simulink model "GenOptRockerMomtryDisHndlr"  (R2017b)
settings: configuration reference "JD_ConfigsetAUTOSARMulti10msec" (kept outside this file)
values from neighbouring files (symbols this model uses):
  EolDurnLong = AUTOSAR.Parameter    [GenOptRockerMomtryDisHndlr_DD.m]
  EolDurnRetain = AUTOSAR.Parameter    [GORMDH_DD.m]
  EolDurnSho = AUTOSAR.Parameter    [GenOptRockerMomtryDisHndlr_DD.m]
  RMI_Error = Simulink.Parameter    [GORMDH_DD.m]
  Transition_Add = Simulink.Parameter    [GORMDH_DD.m]
  Transition_Count = Simulink.Parameter    [GORMDH_DD.m]
  Transition_Zero = Simulink.Parameter    [GORMDH_DD.m]
undefined symbols (not defined in the file or in its folder): DiagBool, EnCtrlDisSt, EnCtrlSeln, EnCtrlSts
libraries: simulink x3
settings Model: Creator=KIH3CPW  LastModifiedBy=KIH3CPW
settings ConfigSetRef: SourceLocation=Base Workspace

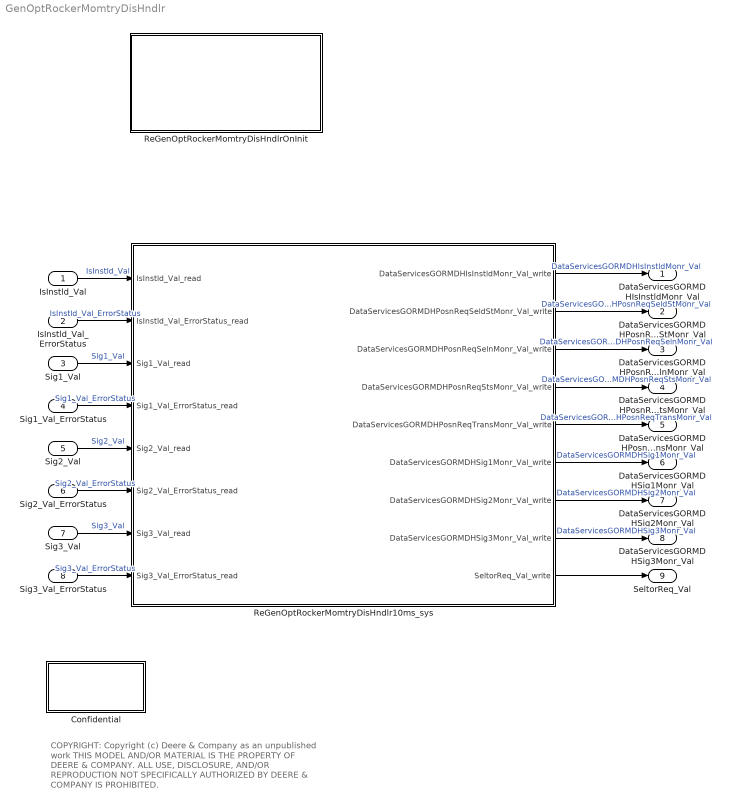
== system GenOptRockerMomtryDisHndlr ==
  note: COPYRIGHT:
      | Copyright (c) Deere & Company as an unpublished work
      | THIS MODEL AND/OR MATERIAL IS THE PROPERTY OF
      | DEERE & COMPANY.  ALL USE, DISCLOSURE, AND/OR
      | REPRODUCTION NOT SPECIFICALLY AUTHORIZED BY
      | DEERE & COMPANY IS PROHIBITED.
  IsInstld_Val : Inport  OutDataTypeStr=Bool  PortDimensions=1
  IsInstld_Val_ErrorStatus : Inport  Port=2  OutDataTypeStr=uint8  PortDimensions=1
  Sig1_Val : Inport  Port=3  OutDataTypeStr=Bool  PortDimensions=1
  Sig1_Val_ErrorStatus : Inport  Port=4  OutDataTypeStr=uint8  PortDimensions=1
  Sig2_Val : Inport  Port=5  OutDataTypeStr=Bool  PortDimensions=1
  Sig2_Val_ErrorStatus : Inport  Port=6  OutDataTypeStr=uint8  PortDimensions=1
  Sig3_Val : Inport  Port=7  OutDataTypeStr=Bool  PortDimensions=1
  Sig3_Val_ErrorStatus : Inport  Port=8  OutDataTypeStr=uint8  PortDimensions=1
  Confidential : Subsystem
      mask Display: image('ConfidentialStamp.jpg')
  ReGenOptRockerMomtryDisHndlr10ms_sys : Subsystem  TreatAsAtomicUnit=on  SystemSampleTime=0.01
  ReGenOptRockerMomtryDisHndlrOnInit : Subsystem
  DataServicesGORMDHIsInstldMonr_Val : Outport  OutDataTypeStr=Enum: DiagBool  PortDimensions=1
  DataServicesGORMDHPosnReqSeldStMonr_Val : Outport  Port=2  OutDataTypeStr=Enum: EnCtrlDisSt  PortDimensions=1
  DataServicesGORMDHPosnReqSelnMonr_Val : Outport  Port=3  OutDataTypeStr=Enum: EnCtrlSeln  PortDimensions=1
  DataServicesGORMDHPosnReqStsMonr_Val : Outport  Port=4  OutDataTypeStr=Enum: EnCtrlSts  PortDimensions=1
  DataServicesGORMDHPosnReqTransMonr_Val : Outport  Port=5  OutDataTypeStr=CntAbsMod  PortDimensions=1
  DataServicesGORMDHSig1Monr_Val : Outport  Port=6  OutDataTypeStr=Enum: DiagBool  PortDimensions=1
  DataServicesGORMDHSig2Monr_Val : Outport  Port=7  OutDataTypeStr=Enum: DiagBool  PortDimensions=1
  DataServicesGORMDHSig3Monr_Val : Outport  Port=8  OutDataTypeStr=Enum: DiagBool  PortDimensions=1
  SeltorReq_Val : Outport  Port=9  OutDataTypeStr=Bus: RecCtrlSelr  PortDimensions=1  BusOutputAsStruct=on
  wires:
  IsInstld_Val/1 -> ReGenOptRockerMomtryDisHndlr10ms_sys/1(IsInstld_Val_read)  "IsInstld_Val"
  IsInstld_Val_ErrorStatus/1 -> ReGenOptRockerMomtryDisHndlr10ms_sys/2(IsInstld_Val_ErrorStatus_read)  "IsInstld_Val_ErrorStatus"
  Sig1_Val/1 -> ReGenOptRockerMomtryDisHndlr10ms_sys/3(Sig1_Val_read)  "Sig1_Val"
  Sig1_Val_ErrorStatus/1 -> ReGenOptRockerMomtryDisHndlr10ms_sys/4(Sig1_Val_ErrorStatus_read)  "Sig1_Val_ErrorStatus"
  Sig2_Val/1 -> ReGenOptRockerMomtryDisHndlr10ms_sys/5(Sig2_Val_read)  "Sig2_Val"
  Sig2_Val_ErrorStatus/1 -> ReGenOptRockerMomtryDisHndlr10ms_sys/6(Sig2_Val_ErrorStatus_read)  "Sig2_Val_ErrorStatus"
  Sig3_Val/1 -> ReGenOptRockerMomtryDisHndlr10ms_sys/7(Sig3_Val_read)  "Sig3_Val"
  Sig3_Val_ErrorStatus/1 -> ReGenOptRockerMomtryDisHndlr10ms_sys/8(Sig3_Val_ErrorStatus_read)  "Sig3_Val_ErrorStatus"
  ReGenOptRockerMomtryDisHndlr10ms_sys/1(DataServicesGORMDHIsInstldMonr_Val_write) -> DataServicesGORMDHIsInstldMonr_Val/1  "DataServicesGORMDHIsInstldMonr_Val"
  ReGenOptRockerMomtryDisHndlr10ms_sys/2(DataServicesGORMDHPosnReqSeldStMonr_Val_write) -> DataServicesGORMDHPosnReqSeldStMonr_Val/1  "DataServicesGORMDHPosnReqSeldStMonr_Val"
  ReGenOptRockerMomtryDisHndlr10ms_sys/3(DataServicesGORMDHPosnReqSelnMonr_Val_write) -> DataServicesGORMDHPosnReqSelnMonr_Val/1  "DataServicesGORMDHPosnReqSelnMonr_Val"
  ReGenOptRockerMomtryDisHndlr10ms_sys/4(DataServicesGORMDHPosnReqStsMonr_Val_write) -> DataServicesGORMDHPosnReqStsMonr_Val/1  "DataServicesGORMDHPosnReqStsMonr_Val"
  ReGenOptRockerMomtryDisHndlr10ms_sys/5(DataServicesGORMDHPosnReqTransMonr_Val_write) -> DataServicesGORMDHPosnReqTransMonr_Val/1  "DataServicesGORMDHPosnReqTransMonr_Val"
  ReGenOptRockerMomtryDisHndlr10ms_sys/6(DataServicesGORMDHSig1Monr_Val_write) -> DataServicesGORMDHSig1Monr_Val/1  "DataServicesGORMDHSig1Monr_Val"
  ReGenOptRockerMomtryDisHndlr10ms_sys/7(DataServicesGORMDHSig2Monr_Val_write) -> DataServicesGORMDHSig2Monr_Val/1  "DataServicesGORMDHSig2Monr_Val"
  ReGenOptRockerMomtryDisHndlr10ms_sys/8(DataServicesGORMDHSig3Monr_Val_write) -> DataServicesGORMDHSig3Monr_Val/1  "DataServicesGORMDHSig3Monr_Val"
  ReGenOptRockerMomtryDisHndlr10ms_sys/9(SeltorReq_Val_write) -> SeltorReq_Val/1

== system GenOptRockerMomtryDisHndlr/Confidential ==

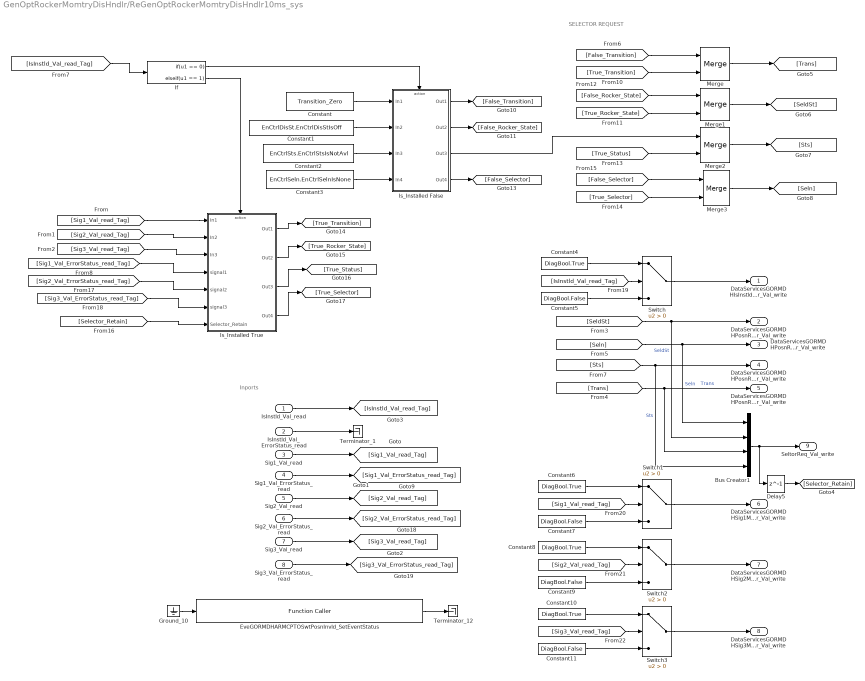
== system GenOptRockerMomtryDisHndlr/ReGenOptRockerMomtryDisHndlr10ms_sys ==
  note: SELECTOR REQUEST
  note: Inports
  IsInstld_Val_read : Inport
  IsInstld_Val_ErrorStatus_read : Inport  Port=2
  Sig1_Val_read : Inport  Port=3
  Sig1_Val_ErrorStatus_read : Inport  Port=4
  Sig2_Val_read : Inport  Port=5
  Sig2_Val_ErrorStatus_read : Inport  Port=6
  Sig3_Val_read : Inport  Port=7
  Sig3_Val_ErrorStatus_read : Inport  Port=8
  Bus Creator1 : BusCreator  Inputs=4  OutDataTypeStr=Bus: RecCtrlSelr
  Constant : Constant  Value=Transition_Zero  OutDataTypeStr=CntAbsMod
  Constant1 : Constant  Value=EnCtrlDisSt.EnCtrlDisStIsOff
  Constant{4,6,8,10} (4 alike) : Constant  Value=DiagBool.True
  Constant{5,7,9,11} (4 alike) : Constant  Value=DiagBool.False
  Constant2 : Constant  Value=EnCtrlSts.EnCtrlStsIsNotAvl
  Constant3 : Constant  Value=EnCtrlSeln.EnCtrlSelnIsNone
  Delay5 : Delay  DelayLength=1  InitialCondition=0
  EveGORMDHARMCPTOSwtPosnInvld_SetEventStatus : FunctionCaller  Description=API for SWCs to report a monitor result to the Dem.This function is reentrant (for different EventId).This function is not reentrant with the other operations defined in DiagnosticMonitor (for the same EventId)This function is synchronous.  FunctionPrototype=ERR = EveGORMDHARMCPTOSwtPosnInvld_SetEventStatus(EventStatus)  InputArgumentSpecifications=Dem_EventStatusType.DEM_EVENT_STATUS_PASSED  OutputArgumentSpecifications=P_Std_ReturnType
  Ground_10 : Ground
  If : If  IfExpression=u1 == 0  ElseIfExpressions=u1 == 1  ShowElse=off
  Is_Installed False : Subsystem  TreatAsAtomicUnit=on
  Is_Installed True : Subsystem  TreatAsAtomicUnit=on
  Merge{,1..3} (4 alike) : Merge
  Switch{,1..3} (4 alike) : Switch  Criteria=u2 > Threshold
  Terminator_1 : Terminator
  Terminator_12 : Terminator
  DataServicesGORMDHIsInstldMonr_Val_write : Outport
  DataServicesGORMDHPosnReqSeldStMonr_Val_write : Outport  Port=2
  DataServicesGORMDHPosnReqSelnMonr_Val_write : Outport  Port=3
  DataServicesGORMDHPosnReqStsMonr_Val_write : Outport  Port=4
  DataServicesGORMDHPosnReqTransMonr_Val_write : Outport  Port=5
  DataServicesGORMDHSig1Monr_Val_write : Outport  Port=6
  DataServicesGORMDHSig2Monr_Val_write : Outport  Port=7
  DataServicesGORMDHSig3Monr_Val_write : Outport  Port=8
  SeltorReq_Val_write : Outport  Port=9  OutDataTypeStr=Bus: RecCtrlSelr
  wires:
  Switch/1 -> DataServicesGORMDHIsInstldMonr_Val_write/1
  Switch1/1 -> DataServicesGORMDHSig1Monr_Val_write/1
  Switch2/1 -> DataServicesGORMDHSig2Monr_Val_write/1
  Switch3/1 -> DataServicesGORMDHSig3Monr_Val_write/1
  IsInstld_Val_ErrorStatus_read/1 -> Terminator_1/1
  Sig1_Val_read/1 -> [Sig1_Val_read_Tag]
  Sig1_Val_ErrorStatus_read/1 -> [Sig1_Val_ErrorStatus_read_Tag]
  Sig2_Val_read/1 -> [Sig2_Val_read_Tag]
  Sig2_Val_ErrorStatus_read/1 -> [Sig2_Val_ErrorStatus_read_Tag]
  Sig3_Val_read/1 -> [Sig3_Val_read_Tag]
  Sig3_Val_ErrorStatus_read/1 -> [Sig3_Val_ErrorStatus_read_Tag]
  Ground_10/1 -> EveGORMDHARMCPTOSwtPosnInvld_SetEventStatus/1
  EveGORMDHARMCPTOSwtPosnInvld_SetEventStatus/1 -> Terminator_12/1
  [Sig1_Val_read_Tag] -> Is_Installed True/1(In1)
  [Sig2_Val_read_Tag] -> Is_Installed True/2(In2)
  [Sig3_Val_read_Tag] -> Is_Installed True/3(In3)
  IsInstld_Val_read/1 -> [IsInstld_Val_read_Tag]
  Merge/1 -> [Trans]
  Merge1/1 -> [SeldSt]
  Merge2/1 -> [Sts]
  Is_Installed True/1(Out1) -> [True_Transition]
  Is_Installed True/2(Out2) -> [True_Rocker_State]
  Is_Installed True/4(Out4) -> [True_Selector]
  [False_Transition] -> Merge/1
  [False_Rocker_State] -> Merge1/1
  [True_Rocker_State] -> Merge1/2
  Is_Installed False/3(Out3) -> Merge2/1
  [False_Selector] -> Merge3/1
  [True_Selector] -> Merge3/2
  [IsInstld_Val_read_Tag] -> If/1
  If/1 -> Is_Installed False/Action
  Constant/1 -> Is_Installed False/1(In1)
  Constant1/1 -> Is_Installed False/2(In2)
  Constant2/1 -> Is_Installed False/3(In3)
  Constant3/1 -> Is_Installed False/4(In4)
  Is_Installed False/1(Out1) -> [False_Transition]
  Is_Installed False/2(Out2) -> [False_Rocker_State]
  Is_Installed False/4(Out4) -> [False_Selector]
  If/2 -> Is_Installed True/Action
  Constant4/1 -> Switch/1
  Constant5/1 -> Switch/3
  [IsInstld_Val_read_Tag] -> Switch/2
  [Sig1_Val_read_Tag] -> Switch1/2
  Constant7/1 -> Switch1/3
  Constant6/1 -> Switch1/1
  [Sig2_Val_read_Tag] -> Switch2/2
  Constant8/1 -> Switch2/1
  Constant9/1 -> Switch2/3
  [Sig3_Val_read_Tag] -> Switch3/2
  Constant10/1 -> Switch3/1
  Constant11/1 -> Switch3/3
  Merge3/1 -> [Seln]
  Delay5/1 -> [Selector_Retain]
  Bus Creator1/1 -> SeltorReq_Val_write/1, Delay5/1
  [Sts] -> Bus Creator1/4, DataServicesGORMDHPosnReqStsMonr_Val_write/1  "Sts"
  [Trans] -> Bus Creator1/3, DataServicesGORMDHPosnReqTransMonr_Val_write/1  "Trans"
  [Seln] -> Bus Creator1/1, DataServicesGORMDHPosnReqSelnMonr_Val_write/1  "Seln"
  [SeldSt] -> Bus Creator1/2, DataServicesGORMDHPosnReqSeldStMonr_Val_write/1  "SeldSt"
  [Sig1_Val_ErrorStatus_read_Tag] -> Is_Installed True/4(signal1)
  [Sig3_Val_ErrorStatus_read_Tag] -> Is_Installed True/6("signal3 ")
  Is_Installed True/3(Out3) -> [True_Status]
  [True_Status] -> Merge2/2
  [Selector_Retain] -> Is_Installed True/7(Selector_Retain)
  [Sig2_Val_ErrorStatus_read_Tag] -> Is_Installed True/5(signal2)
  [True_Transition] -> Merge/2

== system GenOptRockerMomtryDisHndlr/ReGenOptRockerMomtryDisHndlrOnInit ==
  Event Listener : EventListener  EventType=Initialize  EventName=reset  VariantControl=Variant

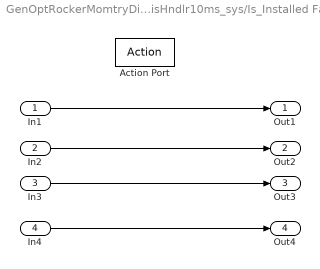
== system GenOptRockerMomtryDisHndlr/ReGenOptRockerMomtryDisHndlr10ms_sys/Is_Installed False ==
  In1 : Inport
  In2 : Inport  Port=2
  In3 : Inport  Port=3
  In4 : Inport  Port=4
  Action Port : ActionPort  ActionType=then
  Out1 : Outport
  Out2 : Outport  Port=2
  Out3 : Outport  Port=3
  Out4 : Outport  Port=4
  wires:
  In1/1 -> Out1/1
  In4/1 -> Out4/1
  In3/1 -> Out3/1
  In2/1 -> Out2/1

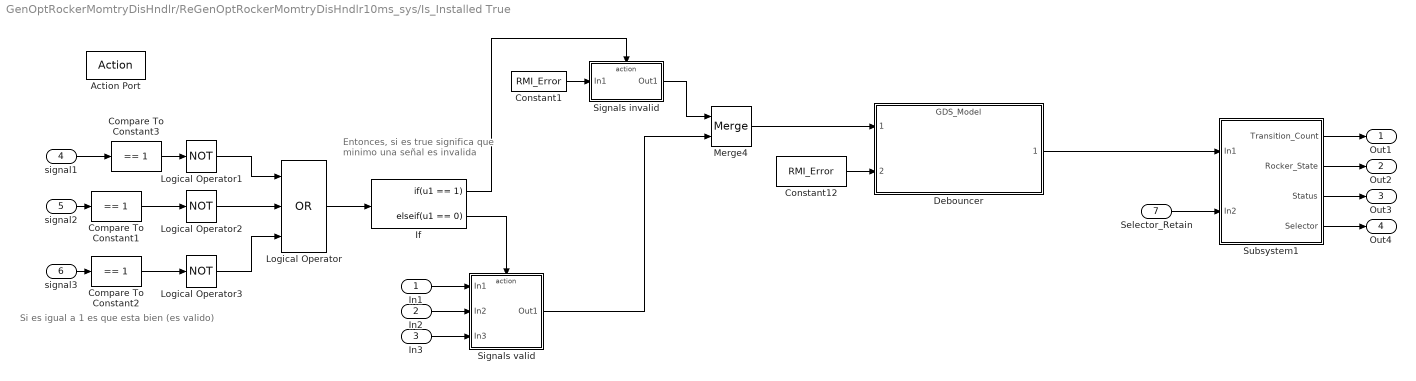
== system GenOptRockerMomtryDisHndlr/ReGenOptRockerMomtryDisHndlr10ms_sys/Is_Installed True ==
  note: Si es igual a 1 es que esta bien (es valido)
  note: Entonces, si es true significa que minimo una señal es invalida
  In1 : Inport
  In2 : Inport  Port=2
  In3 : Inport  Port=3
  signal1 : Inport  Port=4
  signal2 : Inport  Port=5
  "signal3 " : Inport  Port=6
  Selector_Retain : Inport  Port=7
  Action Port : ActionPort  ActionType=elseif
  Compare To Constant1 : simulink/Logic and Bit Operations/Compare To Constant  relop===  const=1  OutDataTypeStr=boolean
  Compare To Constant2 : simulink/Logic and Bit Operations/Compare To Constant  relop===  const=1  OutDataTypeStr=boolean
  Compare To Constant3 : simulink/Logic and Bit Operations/Compare To Constant  relop===  const=1  OutDataTypeStr=boolean
  Constant1 : Constant  Value=RMI_Error
  Constant12 : Constant  Value=RMI_Error
  "Debouncer " : ModelReference  ModelNameDialog=GDS_Model.slx  SimulationMode=Normal  ModelReferenceVersion=1.8
  If : If  IfExpression=u1 == 1  ElseIfExpressions=u1 == 0  ShowElse=off
  Logical Operator : Logic  Operator=OR  Inputs=3  AllPortsSameDT=off  OutDataTypeStr=boolean
  Logical Operator1 : Logic  Operator=NOT  AllPortsSameDT=off  OutDataTypeStr=boolean
  Logical Operator2 : Logic  Operator=NOT  AllPortsSameDT=off  OutDataTypeStr=boolean
  Logical Operator3 : Logic  Operator=NOT  AllPortsSameDT=off  OutDataTypeStr=boolean
  Merge4 : Merge
  Signals invalid : Subsystem  TreatAsAtomicUnit=on
  Signals valid : Subsystem  TreatAsAtomicUnit=on
  Subsystem1 : Subsystem
  Out1 : Outport
  Out2 : Outport  Port=2
  Out3 : Outport  Port=3
  Out4 : Outport  Port=4
  wires:
  In3/1 -> Signals valid/3(In3)
  In2/1 -> Signals valid/2(In2)
  In1/1 -> Signals valid/1(In1)
  Compare To Constant2/1 -> Logical Operator3/1
  Logical Operator2/1 -> Logical Operator/2
  Logical Operator/1 -> If/1
  Logical Operator3/1 -> Logical Operator/3
  Compare To Constant3/1 -> Logical Operator1/1
  signal2/1 -> Compare To Constant1/1
  "signal3 "/1 -> Compare To Constant2/1
  Logical Operator1/1 -> Logical Operator/1
  Compare To Constant1/1 -> Logical Operator2/1
  signal1/1 -> Compare To Constant3/1
  Merge4/1 -> "Debouncer "/1
  Selector_Retain/1 -> Subsystem1/2(In2)
  Constant12/1 -> "Debouncer "/2
  "Debouncer "/1 -> Subsystem1/1(In1)
  Subsystem1/1(Transition_Count) -> Out1/1
  Subsystem1/2(Rocker_State) -> Out2/1
  Subsystem1/3(Status) -> Out3/1
  Subsystem1/4(Selector) -> Out4/1
  If/2 -> Signals valid/Action
  Signals valid/1(Out1) -> Merge4/2
  If/1 -> Signals invalid/Action
  Constant1/1 -> Signals invalid/1(In1)
  Signals invalid/1(Out1) -> Merge4/1

== system GenOptRockerMomtryDisHndlr/ReGenOptRockerMomtryDisHndlr10ms_sys/Is_Installed True/Signals invalid ==
  In1 : Inport
  Action Port : ActionPort  ActionType=then
  Out1 : Outport
  wires:
  In1/1 -> Out1/1

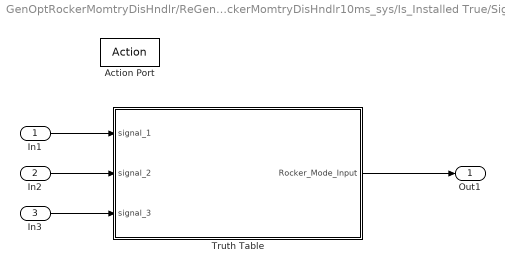
== system GenOptRockerMomtryDisHndlr/ReGenOptRockerMomtryDisHndlr10ms_sys/Is_Installed True/Signals valid ==
  In1 : Inport
  In2 : Inport  Port=2
  In3 : Inport  Port=3
  Action Port : ActionPort  ActionType=elseif
  Truth Table : Truth Table  TreatAsAtomicUnit=on
  Out1 : Outport
  wires:
  In3/1 -> Truth Table/3(signal_3)
  In2/1 -> Truth Table/2(signal_2)
  In1/1 -> Truth Table/1(signal_1)
  Truth Table/1(Rocker_Mode_Input) -> Out1/1

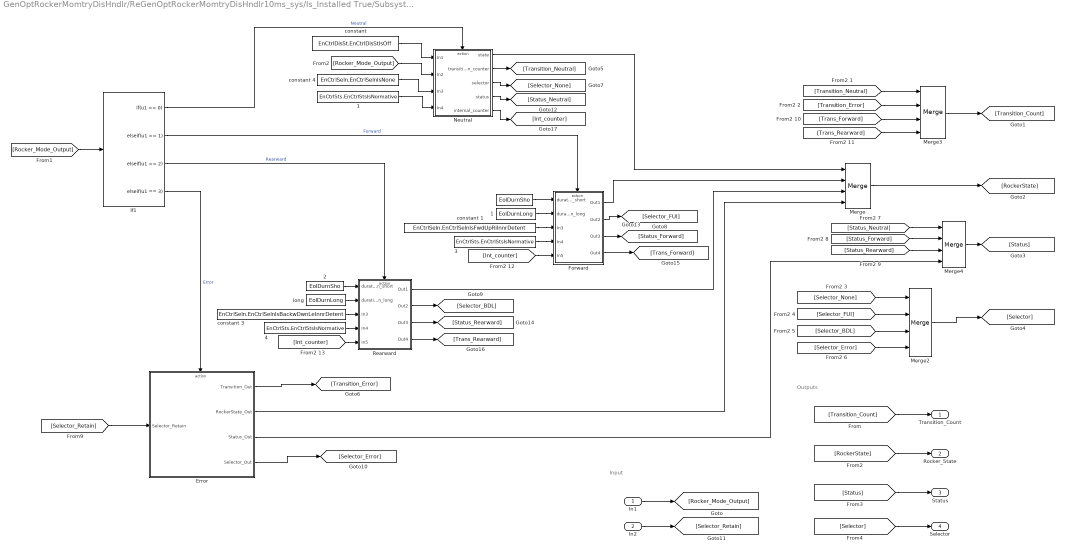
== system GenOptRockerMomtryDisHndlr/ReGenOptRockerMomtryDisHndlr10ms_sys/Is_Installed True/Subsystem1 ==
  note: Outputs
  note: Input
  In1 : Inport
  In2 : Inport  Port=2
  " " : Constant  Value=EolDurnSho
  " 1" : Constant  Value=EolDurnLong
  " 2" : Constant  Value=EolDurnSho
  1 : Constant  Value=EnCtrlSts.EnCtrlStsIsNormative
  3 : Constant  Value=EnCtrlSts.EnCtrlStsIsNormative
  4 : Constant  Value=EnCtrlSts.EnCtrlStsIsNormative
  Error : Subsystem  TreatAsAtomicUnit=on
  Forward : Subsystem  TreatAsAtomicUnit=on
  If1 : If  IfExpression=u1 == 0  ElseIfExpressions=u1 == 1, u1 == 2, u1 == 3  ShowElse=off
  Merge{,2..4} (4 alike) : Merge  Inputs=4
  Neutral : Subsystem  TreatAsAtomicUnit=on
  Rearward : Subsystem  TreatAsAtomicUnit=on
  "constant " : Constant  Value=EnCtrlDisSt.EnCtrlDisStIsOff
  constant 1 : Constant  Value=EnCtrlSeln.EnCtrlSelnIsFwdUpRiInnrDetent
  constant 3 : Constant  Value=EnCtrlSeln.EnCtrlSelnIsBackwDwnLeInnrDetent
  constant 4 : Constant  Value=EnCtrlSeln.EnCtrlSelnIsNone
  long : Constant  Value=EolDurnLong
  Transition_Count : Outport
  Rocker_State : Outport  Port=2
  Status : Outport  Port=3
  Selector : Outport  Port=4
  wires:
  If1/4 -> Error/Action  "Error"
  " "/1 -> Forward/1(duration_short)
  Merge/1 -> [RockerState]
  Neutral/1(state) -> Merge/1
  [Rocker_Mode_Output] -> Neutral/2(In2)
  If1/1 -> Neutral/Action  "Neutral"
  "constant "/1 -> Neutral/1(In1)
  constant 3/1 -> Rearward/3(In3)
  Forward/1(Out1) -> Merge/2
  If1/3 -> Rearward/Action  "Rearward"
  [Rocker_Mode_Output] -> If1/1
  In1/1 -> [Rocker_Mode_Output]
  [Transition_Count] -> Transition_Count/1
  [RockerState] -> Rocker_State/1
  [Status] -> Status/1
  Merge2/1 -> [Selector]
  [Selector] -> Selector/1
  Merge3/1 -> [Transition_Count]
  Merge4/1 -> [Status]
  Error/3(Status_Out) -> Merge4/4
  " 1"/1 -> Forward/2(duration_long)
  constant 4/1 -> Neutral/3(In3)
  constant 1/1 -> Forward/3(In3)
  If1/2 -> Forward/Action  "Forward"
  " 2"/1 -> Rearward/1(duration_short)
  long/1 -> Rearward/2(duration_long)
  Neutral/2(transition_counter) -> [Transition_Neutral]
  Error/1(Transition_Out) -> [Transition_Error]
  [Transition_Error] -> Merge3/2
  [Transition_Neutral] -> Merge3/1
  Neutral/3(selector) -> [Selector_None]
  Forward/2(Out2) -> [Selector_FUI]
  Rearward/2(Out2) -> [Selector_BDL]
  Error/4(Selector_Out) -> [Selector_Error]
  [Selector_None] -> Merge2/1
  [Selector_FUI] -> Merge2/2
  [Selector_BDL] -> Merge2/3
  [Selector_Error] -> Merge2/4
  Rearward/1(Out1) -> Merge/3
  Error/2(RockerState_Out) -> Merge/4
  In2/1 -> [Selector_Retain]
  1/1 -> Neutral/4(In4)
  Neutral/4(status) -> [Status_Neutral]
  3/1 -> Forward/4(In4)
  Forward/3(Out3) -> [Status_Forward]
  4/1 -> Rearward/4(In4)
  Rearward/3(Out3) -> [Status_Rearward]
  [Status_Neutral] -> Merge4/1
  [Status_Forward] -> Merge4/2
  [Status_Rearward] -> Merge4/3
  [Selector_Retain] -> Error/1(Selector_Retain)
  Forward/4(Out4) -> [Trans_Forward]
  [Trans_Forward] -> Merge3/3
  [Trans_Rearward] -> Merge3/4
  [Int_counter] -> Rearward/5(In5)
  Rearward/4(Out4) -> [Trans_Rearward]
  [Int_counter] -> Forward/5(In5)
  Neutral/5(internal_counter) -> [Int_counter]

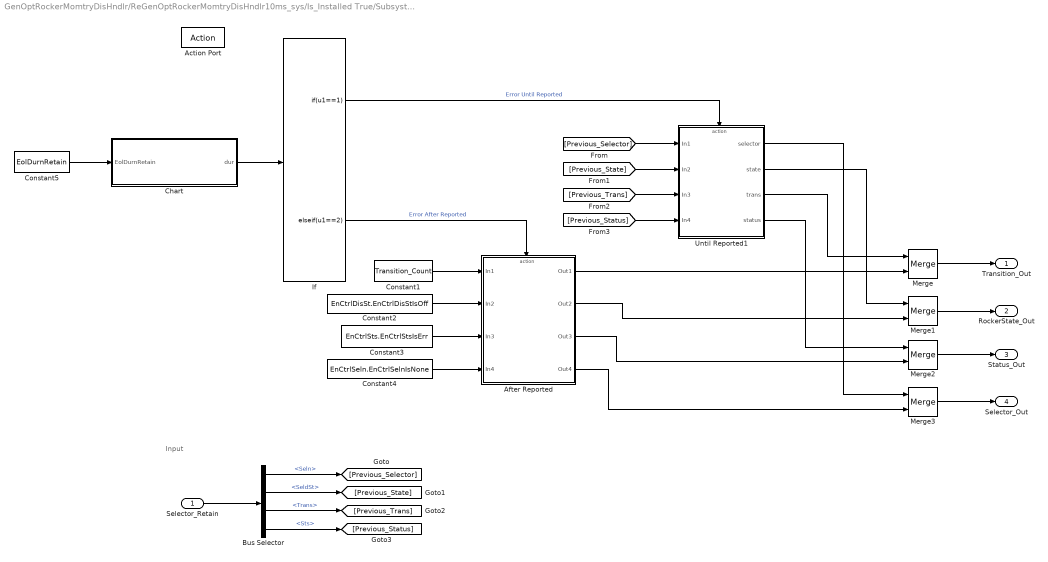
== system GenOptRockerMomtryDisHndlr/ReGenOptRockerMomtryDisHndlr10ms_sys/Is_Installed True/Subsystem1/Error ==
  note: Input
  Selector_Retain : Inport
  Action Port : ActionPort  ActionType=elseif
  After Reported : Subsystem  TreatAsAtomicUnit=on
  Bus Selector : BusSelector  OutputSignals=Seln,SeldSt,Trans,Sts
  Chart : Stateflow chart  TreatAsAtomicUnit=on
  Constant1 : Constant  Value=Transition_Count
  Constant2 : Constant  Value=EnCtrlDisSt.EnCtrlDisStIsOff
  Constant3 : Constant  Value=EnCtrlSts.EnCtrlStsIsErr
  Constant4 : Constant  Value=EnCtrlSeln.EnCtrlSelnIsNone
  Constant5 : Constant  Value=EolDurnRetain
  If : If  IfExpression=u1==1  ElseIfExpressions=u1==2  ShowElse=off
  Merge{,1..3} (4 alike) : Merge
  Until Reported1 : Subsystem  TreatAsAtomicUnit=on
  Transition_Out : Outport
  RockerState_Out : Outport  Port=2
  Status_Out : Outport  Port=3
  Selector_Out : Outport  Port=4
  wires:
  Chart/1(dur) -> If/1
  Constant5/1 -> Chart/1(EolDurnRetain)
  After Reported/3(Out3) -> Merge2/2
  After Reported/2(Out2) -> Merge1/2
  After Reported/4(Out4) -> Merge3/2
  Constant3/1 -> After Reported/3(In3)
  Merge1/1 -> RockerState_Out/1
  After Reported/1(Out1) -> Merge/2
  Constant1/1 -> After Reported/1(In1)
  If/2 -> After Reported/Action  "Error After Reported"
  Merge3/1 -> Selector_Out/1
  Constant4/1 -> After Reported/4(In4)
  If/1 -> Until Reported1/Action  "Error Until Reported"
  Until Reported1/2(state) -> Merge1/1
  Merge/1 -> Transition_Out/1
  Merge2/1 -> Status_Out/1
  Constant2/1 -> After Reported/2(In2)
  Until Reported1/1(selector) -> Merge3/1
  Until Reported1/3(trans) -> Merge/1
  Until Reported1/4(status) -> Merge2/1
  Selector_Retain/1 -> Bus Selector/1
  Bus Selector/1 -> [Previous_Selector]  "<Seln>"
  Bus Selector/2 -> [Previous_State]  "<SeldSt>"
  Bus Selector/3 -> [Previous_Trans]  "<Trans>"
  Bus Selector/4 -> [Previous_Status]  "<Sts>"
  [Previous_Selector] -> Until Reported1/1(In1)
  [Previous_State] -> Until Reported1/2(In2)
  [Previous_Trans] -> Until Reported1/3(In3)
  [Previous_Status] -> Until Reported1/4(In4)

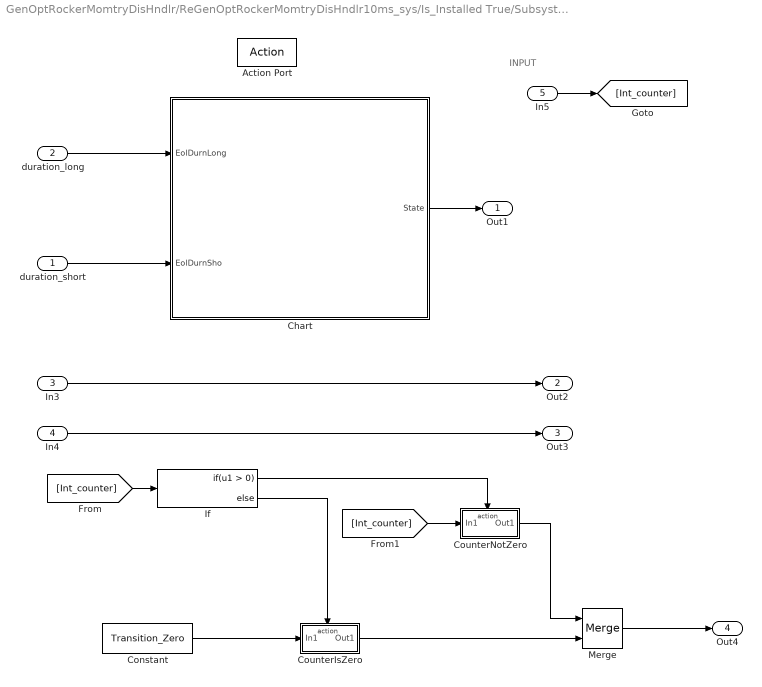
== system GenOptRockerMomtryDisHndlr/ReGenOptRockerMomtryDisHndlr10ms_sys/Is_Installed True/Subsystem1/Forward ==
  note: INPUT
  duration_short : Inport
  duration_long : Inport  Port=2
  In3 : Inport  Port=3
  In4 : Inport  Port=4
  In5 : Inport  Port=5  OutDataTypeStr=CntAbsMod
  Action Port : ActionPort  ActionType=elseif
  Chart : Stateflow chart  TreatAsAtomicUnit=on
  Constant : Constant  Value=Transition_Zero  OutDataTypeStr=CntAbsMod
  CounterIsZero : Subsystem  TreatAsAtomicUnit=on
  CounterNotZero : Subsystem  TreatAsAtomicUnit=on
  If : If
  Merge : Merge
  Out1 : Outport
  Out2 : Outport  Port=2
  Out3 : Outport  Port=3
  Out4 : Outport  Port=4  OutDataTypeStr=CntAbsMod
  wires:
  In3/1 -> Out2/1
  Chart/1(State) -> Out1/1
  In4/1 -> Out3/1
  duration_long/1 -> Chart/1(EolDurnLong)
  duration_short/1 -> Chart/2(EolDurnSho)
  In5/1 -> [Int_counter]
  [Int_counter] -> If/1
  If/1 -> CounterNotZero/Action
  If/2 -> CounterIsZero/Action
  [Int_counter] -> CounterNotZero/1(In1)
  Constant/1 -> CounterIsZero/1(In1)
  CounterIsZero/1(Out1) -> Merge/2
  Merge/1 -> Out4/1
  CounterNotZero/1(Out1) -> Merge/1

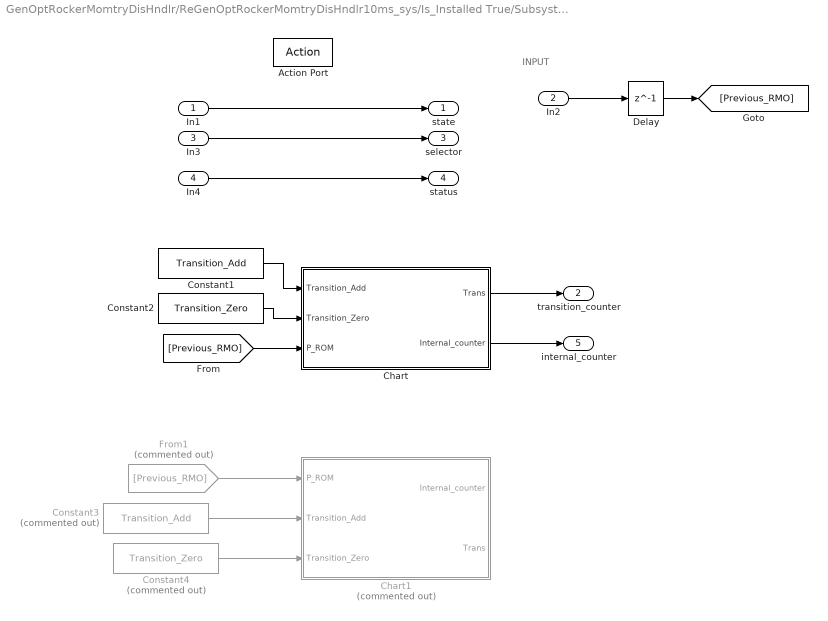
== system GenOptRockerMomtryDisHndlr/ReGenOptRockerMomtryDisHndlr10ms_sys/Is_Installed True/Subsystem1/Neutral ==
  note: INPUT
  In1 : Inport
  In2 : Inport  Port=2
  In3 : Inport  Port=3
  In4 : Inport  Port=4
  Action Port : ActionPort  ActionType=then
  Chart : Stateflow chart  TreatAsAtomicUnit=on
  Chart1 : Stateflow chart  Commented=on  TreatAsAtomicUnit=on
  Constant1 : Constant  Value=Transition_Add
  Constant2 : Constant  Value=Transition_Zero
  Constant3 : Constant  Commented=on  Value=Transition_Add
  Constant4 : Constant  Commented=on  Value=Transition_Zero
  Delay : Delay  DelayLength=1  InitialCondition=0
  From1 : From  Commented=on  GotoTag=Previous_RMO
  state : Outport
  transition_counter : Outport  Port=2  OutDataTypeStr=CntAbsMod
  selector : Outport  Port=3
  status : Outport  Port=4
  internal_counter : Outport  Port=5  OutDataTypeStr=CntAbsMod
  wires:
  In1/1 -> state/1
  Delay/1 -> [Previous_RMO]
  In2/1 -> Delay/1
  In3/1 -> selector/1
  In4/1 -> status/1
  From1/1 -> Chart1/1(P_ROM)
  Constant4/1 -> Chart1/3(Transition_Zero)
  Constant3/1 -> Chart1/2(Transition_Add)
  Constant1/1 -> Chart/1(Transition_Add)
  Constant2/1 -> Chart/2(Transition_Zero)
  [Previous_RMO] -> Chart/3(P_ROM)
  Chart/2(Internal_counter) -> internal_counter/1
  Chart/1(Trans) -> transition_counter/1

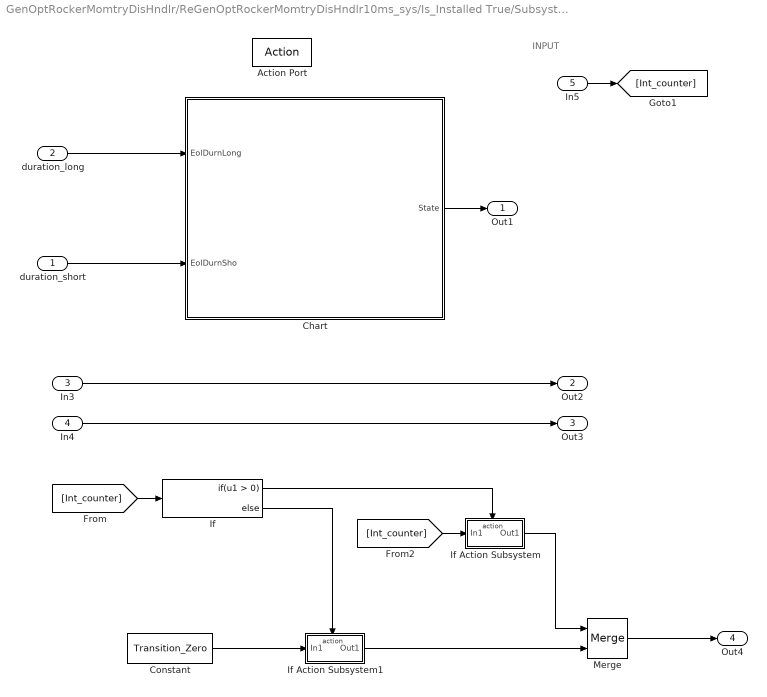
== system GenOptRockerMomtryDisHndlr/ReGenOptRockerMomtryDisHndlr10ms_sys/Is_Installed True/Subsystem1/Rearward ==
  note: INPUT
  duration_short : Inport
  duration_long : Inport  Port=2
  In3 : Inport  Port=3
  In4 : Inport  Port=4
  In5 : Inport  Port=5
  Action Port : ActionPort  ActionType=elseif
  Chart : Stateflow chart  TreatAsAtomicUnit=on
  Constant : Constant  Value=Transition_Zero  OutDataTypeStr=CntAbsMod
  If : If
  If Action Subsystem : Subsystem  TreatAsAtomicUnit=on
  If Action Subsystem1 : Subsystem  TreatAsAtomicUnit=on
  Merge : Merge
  Out1 : Outport
  Out2 : Outport  Port=2
  Out3 : Outport  Port=3
  Out4 : Outport  Port=4  OutDataTypeStr=CntAbsMod
  wires:
  In3/1 -> Out2/1
  Chart/1(State) -> Out1/1
  In4/1 -> Out3/1
  duration_short/1 -> Chart/2(EolDurnSho)
  duration_long/1 -> Chart/1(EolDurnLong)
  If/1 -> If Action Subsystem/Action
  If/2 -> If Action Subsystem1/Action
  Constant/1 -> If Action Subsystem1/1(In1)
  [Int_counter] -> If/1
  [Int_counter] -> If Action Subsystem/1(In1)
  Merge/1 -> Out4/1
  If Action Subsystem/1(Out1) -> Merge/1
  If Action Subsystem1/1(Out1) -> Merge/2
  In5/1 -> [Int_counter]

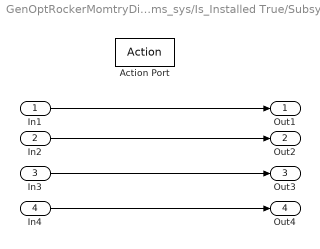
== system GenOptRockerMomtryDisHndlr/ReGenOptRockerMomtryDisHndlr10ms_sys/Is_Installed True/Subsystem1/Error/After Reported ==
  In1 : Inport
  In2 : Inport  Port=2
  In3 : Inport  Port=3
  In4 : Inport  Port=4
  Action Port : ActionPort  ActionType=elseif
  Out1 : Outport
  Out2 : Outport  Port=2
  Out3 : Outport  Port=3
  Out4 : Outport  Port=4
  wires:
  In1/1 -> Out1/1
  In2/1 -> Out2/1
  In3/1 -> Out3/1
  In4/1 -> Out4/1

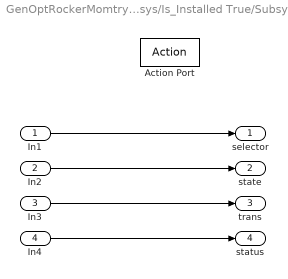
== system GenOptRockerMomtryDisHndlr/ReGenOptRockerMomtryDisHndlr10ms_sys/Is_Installed True/Subsystem1/Error/Until Reported1 ==
  In1 : Inport  OutDataTypeStr=Enum: EnCtrlSeln
  In2 : Inport  Port=2  OutDataTypeStr=Enum: EnCtrlDisSt
  In3 : Inport  Port=3  OutDataTypeStr=CntAbsMod
  In4 : Inport  Port=4  OutDataTypeStr=Enum: EnCtrlSts
  Action Port : ActionPort  ActionType=then
  selector : Outport  OutDataTypeStr=Enum: EnCtrlSeln
  state : Outport  Port=2  OutDataTypeStr=Enum: EnCtrlDisSt
  trans : Outport  Port=3  OutDataTypeStr=CntAbsMod
  status : Outport  Port=4  OutDataTypeStr=Enum: EnCtrlSts
  wires:
  In1/1 -> selector/1
  In2/1 -> state/1
  In3/1 -> trans/1
  In4/1 -> status/1

== system GenOptRockerMomtryDisHndlr/ReGenOptRockerMomtryDisHndlr10ms_sys/Is_Installed True/Subsystem1/Forward/CounterIsZero ==
  In1 : Inport  OutDataTypeStr=CntAbsMod
  Action Port : ActionPort  ActionType=else
  Out1 : Outport  OutDataTypeStr=CntAbsMod
  wires:
  In1/1 -> Out1/1

== system GenOptRockerMomtryDisHndlr/ReGenOptRockerMomtryDisHndlr10ms_sys/Is_Installed True/Subsystem1/Forward/CounterNotZero ==
  In1 : Inport  OutDataTypeStr=CntAbsMod
  Action Port : ActionPort  ActionType=then
  Out1 : Outport  OutDataTypeStr=CntAbsMod
  wires:
  In1/1 -> Out1/1

== system GenOptRockerMomtryDisHndlr/ReGenOptRockerMomtryDisHndlr10ms_sys/Is_Installed True/Subsystem1/Rearward/If Action Subsystem ==
  In1 : Inport
  Action Port : ActionPort  ActionType=then
  Out1 : Outport
  wires:
  In1/1 -> Out1/1

== system GenOptRockerMomtryDisHndlr/ReGenOptRockerMomtryDisHndlr10ms_sys/Is_Installed True/Subsystem1/Rearward/If Action Subsystem1 ==
  In1 : Inport  OutDataTypeStr=CntAbsMod
  Action Port : ActionPort  ActionType=else
  Out1 : Outport  OutDataTypeStr=CntAbsMod
  wires:
  In1/1 -> Out1/1

== matlab function GenOptRockerMomtryDisHndlr/ReGenOptRockerMomtryDisHndlr10ms_sys/Is_Installed True/Signals valid/Truth Table ==
  data: signal_1 input boolean; signal_2 input boolean; Rocker_Mode_Input output double; signal_3 input boolean
function Rocker_Mode_Input = fcn(signal_1, signal_2, signal_3)

aVarTruthTableCondition_1 = false;
aVarTruthTableCondition_2 = false;
aVarTruthTableCondition_3 = false;


% Signal 1

aVarTruthTableCondition_1 = logical(signal_1 == 1);

% Signal 2

aVarTruthTableCondition_2 = logical(signal_2 == 1);

% Signal 3

aVarTruthTableCondition_3 = logical(signal_3 == 1);

if (~aVarTruthTableCondition_1 && ~aVarTruthTableCondition_2 && ~aVarTruthTableCondition_3)
    aFcnTruthTableAction_4();
elseif (~aVarTruthTableCondition_1 && ~aVarTruthTableCondition_2 && aVarTruthTableCondition_3)
    aFcnTruthTableAction_1();
elseif (~aVarTruthTableCondition_1 && aVarTruthTableCondition_2 && ~aVarTruthTableCondition_3)
    aFcnTruthTableAction_4();
elseif (~aVarTruthTableCondition_1 && aVarTruthTableCondition_2 && aVarTruthTableCondition_3)
    aFcnTruthTableAction_4();
elseif (aVarTruthTableCondition_1 && ~aVarTruthTableCondition_2 && ~aVarTruthTableCondition_3)
    aFcnTruthTableAction_3();
elseif (aVarTruthTableCondition_1 && ~aVarTruthTableCondition_2 && aVarTruthTableCondition_3)
    aFcnTruthTableAction_4();
elseif (aVarTruthTableCondition_1 && aVarTruthTableCondition_2 && ~aVarTruthTableCondition_3)
    aFcnTruthTableAction_4();
else % Default
    aFcnTruthTableAction_2();
end

function aFcnTruthTableAction_1()

% Neutral

Rocker_Mode_Input = 0;

function aFcnTruthTableAction_2()

% Forward

Rocker_Mode_Input = 1;

function aFcnTruthTableAction_3()

% Rearward

Rocker_Mode_Input = 2;

function aFcnTruthTableAction_4()

% Error

Rocker_Mode_Input = 3;

== stateflow chart GenOptRockerMomtryDisHndlr/ReGenOptRockerMomtryDisHndlr10ms_sys/Is_Installed True/Subsystem1/Forward/Chart ==
  state On
    during:
    State= EnCtrlDisSt.EnCtrlDisStIsOn;
  state HeldShort
    during:
    State= EnCtrlDisSt.EnCtrlDisStIsHoldSho;
  state HeldLong
    during:
    State= EnCtrlDisSt.EnCtrlDisStIsHoldLong;
  (default) -> On
  On -> HeldShort : [after(EolDurnSho, sec) ]
  HeldShort -> HeldLong : [after(EolDurnLong, sec) ]
  data: State output; EolDurnLong input; EolDurnSho input

== stateflow chart GenOptRockerMomtryDisHndlr/ReGenOptRockerMomtryDisHndlr10ms_sys/Is_Installed True/Subsystem1/Neutral/Chart1 ==
  (default) -> (junction 44) : % trans counter
  (junction 44) -> (junction 45) [order 1] : [P_ROM ==1 || P_ROM==2]
  (junction 44) -> (junction 46) [order 2] : {counter= Transition_Zero + counter; Trans= counter; Internal_counter= counter;}
  (junction 45) -> (junction 47) : {counter= Transition_Zero + counter + Transition_Add; Trans= counter; Internal_counter= counter;}
  (junction 47) -> (junction 46)
  (junction 46) -> (junction 48)
  data: P_ROM input; Transition_Add input; Transition_Zero input; Internal_counter output; Trans output; counter local CntAbsMod [0..255] =Transition_Add

== stateflow chart GenOptRockerMomtryDisHndlr/ReGenOptRockerMomtryDisHndlr10ms_sys/Is_Installed True/Subsystem1/Error/Chart ==
  state Error_Until_Reported
    entry:
    dur=1;
  state Error_After_Reported
    entry:
    dur=2;
  (default) -> Error_Until_Reported
  Error_Until_Reported -> Error_After_Reported : [after(EolDurnRetain,sec) ]
  data: EolDurnRetain input; dur output

== stateflow chart GenOptRockerMomtryDisHndlr/ReGenOptRockerMomtryDisHndlr10ms_sys/Is_Installed True/Subsystem1/Rearward/Chart ==
  state On
    during:
    State= EnCtrlDisSt.EnCtrlDisStIsOn;
  state HeldShort
    during:
    State= EnCtrlDisSt.EnCtrlDisStIsHoldSho;
  state HeldLong
    during:
    State= EnCtrlDisSt.EnCtrlDisStIsHoldLong;
  (default) -> On
  On -> HeldShort : [after(EolDurnSho, sec) ]
  HeldShort -> HeldLong : [after(EolDurnLong, sec) ]
  data: State output; EolDurnLong input; EolDurnSho input

== stateflow chart GenOptRockerMomtryDisHndlr/ReGenOptRockerMomtryDisHndlr10ms_sys/Is_Installed True/Subsystem1/Neutral/Chart ==
  state Transition_Increments
    entry:
    counter= counter + Transition_Add+ Transition_Zero;
    Trans= counter;
    Internal_counter= counter;
  state Transition_Same
    entry:
    counter= Transition_Zero + counter;
    Trans= counter;
    Internal_counter=counter;
  state Transition_Increments1
    entry:
    counter= counter + Transition_Add+ Transition_Zero;
    Trans= counter;
    Internal_counter= counter;
  (default) -> Transition_Same
  Transition_Same -> Transition_Increments [order 2] : [P_ROM==1]
  Transition_Increments -> Transition_Same : [P_ROM==0 || P_ROM== 3]
  Transition_Increments1 -> Transition_Same : [P_ROM==0 || P_ROM== 3]
  Transition_Same -> Transition_Increments1 [order 1] : [P_ROM==2]
  data: Trans output; counter local CntAbsMod [0..255] =Transition_Add; Transition_Add input; Transition_Zero input; P_ROM input; Internal_counter output
